simulink model "tutorial_1"  (R2017a)
settings: Solver=VariableStepAuto  StartTime=0.0  StopTime=20.0  MaxStep=0.2  RelTol=1e-3
settings Model: NumberOfSteps=5  SnapshotBufferSize=20  SnapshotInterval=20  Creator=NewOwner  LastModifiedBy=NewOwner

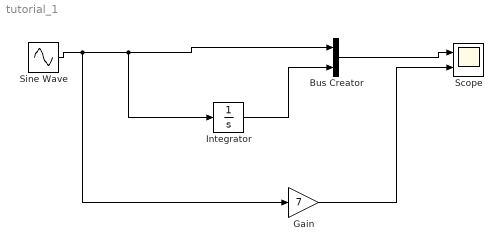
== system tutorial_1 ==
  Bus Creator : BusCreator  Inputs=2
  Gain : Gain  Gain=7
  Integrator : Integrator
  Scope : Scope  NumInputPorts=2
  Sine Wave : Sin  Amplitude=2  SampleTime=0
  wires:
  Sine Wave/1 -> Gain/1, Integrator/1, Bus Creator/1
  Integrator/1 -> Bus Creator/2
  Bus Creator/1 -> Scope/1
  Gain/1 -> Scope/2
